simulink model "EV3_motor_full_model"  (R2022b)
settings: Solver=ode45  StartTime=0.0  StopTime=1.0  RelTol=1e-3
values from neighbouring files (symbols this model uses):
  J = gear_ratio^2 * J_ed    (= 0.0023919264)    [m_for_lab_2.m]
  ke = k_e_static    [m_for_lab_2.m]
  km = ke    [m_for_lab_2.m]
  L = 0.0047    [m_for_lab_2.m]
  R = sum(U .* I) / sum(I.^2)    [m_for_lab_2.m]
undefined symbols (not defined in the file or in its folder): U_sim
settings Model: Creator=Eternal_Core  LastModifiedBy=Eternal_Core

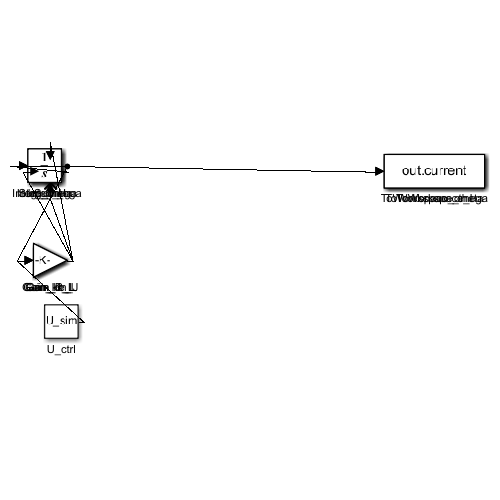
[thumbnail: Simulink's stored preview of the top-level diagram]
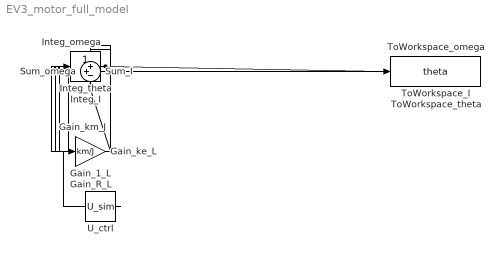
== system EV3_motor_full_model ==
  Gain_1_L : Gain  Gain=1/L
  Gain_R_L : Gain  Gain=R/L
  Gain_ke_L : Gain  Gain=ke/L
  Gain_km_J : Gain  Gain=km/J
  Integ_I : Integrator
  Integ_omega : Integrator
  Integ_theta : Integrator
  Sum_I : Sum  Inputs=++-
  Sum_omega : Sum  Inputs=+-
  ToWorkspace_I : ToWorkspace  VariableName=current  SaveFormat=Structure  SampleTime=-1
  ToWorkspace_omega : ToWorkspace  VariableName=omega  SaveFormat=Structure  SampleTime=-1
  ToWorkspace_theta : ToWorkspace  VariableName=theta  SaveFormat=Structure  SampleTime=-1
  U_ctrl : Constant  Value=U_sim
  wires:
  U_ctrl/1 -> Gain_1_L/1
  Gain_1_L/1 -> Sum_I/1
  Sum_I/1 -> Integ_I/1
  Integ_I/1 -> Gain_km_J/1, Gain_R_L/1, ToWorkspace_I/1
  Gain_km_J/1 -> Sum_omega/1
  Sum_omega/1 -> Integ_omega/1
  Gain_R_L/1 -> Sum_I/3
  Integ_omega/1 -> Gain_ke_L/1, Integ_theta/1, ToWorkspace_omega/1
  Gain_ke_L/1 -> Sum_I/2
  Integ_theta/1 -> ToWorkspace_theta/1
